simulink model "qpsk_transmitter"  (R2013a)
settings: Solver=ode45  StartTime=0.0  StopTime=0.5  RelTol=1e-3
PreLoadFcn:
  | Num
StopFcn:
  | figure(10)
  | hold off
  | plot(i_source(20:end),q_source(20:end),'bo','MarkerFaceColor','b','MarkerSize',6);
  | hold on
  | plot([0 0],[-1.5 1.5],'k:');
  | plot([-1.5 1.5],[0 0],'k:');
  | title('Constellation');
  | xlabel('In Phase');
  | ylabel('Quadrature');
  | axis([-1.5 1.5 -1.5 1.5]);
  | 
  | 
  | figure(11)
  | plot(tx_out);
  | title('Modulated QPSK Signal');
libraries: dsparch4 x2, dspsigops x2
settings Model: Creator=lcrockett  LastModifiedBy=Administrator
settings DataIOCC: SignalLoggingSaveFormat=ModelDataLogs
settings OptimizationCC: ExpressionDepthLimit=2147483647  InitFltsAndDblsToZero=on
settings DebuggingCC: SaveWithParameterizedLinksMsg=none  FcnCallInpInsideContextMsg=UseLocalSettings  StrictBusMsg=Warning
settings GRTTargetCC: TargetFcnLib=ansi_tfl_tmw.mat  CombineOutputUpdateFcns=off  GRTInterface=on

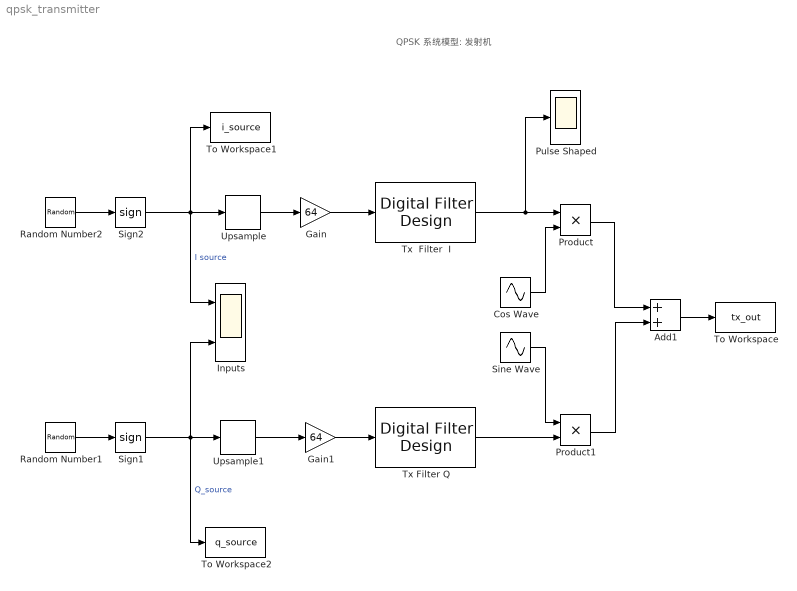
== system qpsk_transmitter ==
  note: QPSK 系统模型: 发射机
  Add1 : Sum
  Cos Wave : Sin  Frequency=(38.4e+3)*2*pi  Phase=pi/2  SampleTime=1/153.6e+3
  Gain : Gain  Gain=64
  Gain1 : Gain  Gain=64
  Inputs : Scope  NumInputPorts=2
      settings: YMin=-1.2~-1.2  YMax=1.2~1.2
  Product : Product  RndMeth=Zero
  Product1 : Product  RndMeth=Zero
  Pulse Shaped : Scope
      settings: YMin=-2  YMax=2
  Random Number1 : RandomNumber  Seed=99  SampleTime=1/2400
  Random Number2 : RandomNumber  Seed=777  SampleTime=1/2400
  Sign1 : Signum
  Sign2 : Signum
  Sine Wave : Sin  Frequency=(38.4e+3)*2*pi  SampleTime=1/153.6e+3
  To Workspace : ToWorkspace  VariableName=tx_out  SampleTime=-1
  To Workspace1 : ToWorkspace  VariableName=i_source  SampleTime=-1
  To Workspace2 : ToWorkspace  VariableName=q_source  SampleTime=-1
  "Tx  Filter  I " : dsparch4/Digital Filter Design  mwdsp_browser_bugfix_var=off
  Tx Filter Q : dsparch4/Digital Filter Design  mwdsp_browser_bugfix_var=off
  Upsample : dspsigops/Upsample  N=64  phase=0  InputProcessing=Inherited (this choice will be removed - see release notes)  RateOptions=Allow multirate processing  ic=0  mode=Unused parameter value
  Upsample1 : dspsigops/Upsample  N=64  phase=0  InputProcessing=Inherited (this choice will be removed - see release notes)  RateOptions=Allow multirate processing  ic=0  mode=Unused parameter value
  wires:
  Sign1/1 -> Upsample1/1, Inputs/2, To Workspace2/1  "Q_source"
  "Tx  Filter  I "/1 -> Product/1, Pulse Shaped/1
  Tx Filter Q/1 -> Product1/2
  Product/1 -> Add1/1
  Product1/1 -> Add1/2
  Add1/1 -> To Workspace/1
  Sign2/1 -> Upsample/1, Inputs/1, To Workspace1/1  "I source"
  Sine Wave/1 -> Product1/1
  Cos Wave/1 -> Product/2
  Gain1/1 -> Tx Filter Q/1
  Random Number2/1 -> Sign2/1
  Random Number1/1 -> Sign1/1
  Gain/1 -> "Tx  Filter  I "/1
  Upsample1/1 -> Gain1/1
  Upsample/1 -> Gain/1
